simulink model "TwoLevel_ThreePhase_SVM_2017b"  (R2017b)
settings: Solver=VariableStepAuto  StartTime=0.0  StopTime=0.1  RelTol=1e-3
StopFcn:
  | Vabc=out.Vabc;
  | Vab=out.Vab;
  | Iabc=out.Iabc;
libraries: powerlib x12
settings Model: Creator=Mehdi  LastModifiedBy=Mehdi
settings DataIOCC: ReturnWorkspaceOutputs=on
settings DebuggingCC: UnconnectedInputMsg=none  UnconnectedOutputMsg=none  UnconnectedLineMsg=none
settings ModelReferenceCC: EnableRefExpFcnMdlSchedulingChecks=off
settings SFSimCC: SimUseLocalCustomCode=on
settings RTWCC: Description=Generic Real-Time Target  RTWUseLocalCustomCode=on
settings CodeAppCC: StateflowObjectComments=on
settings SimscapeCC: SimscapeNormalizeSystem=off

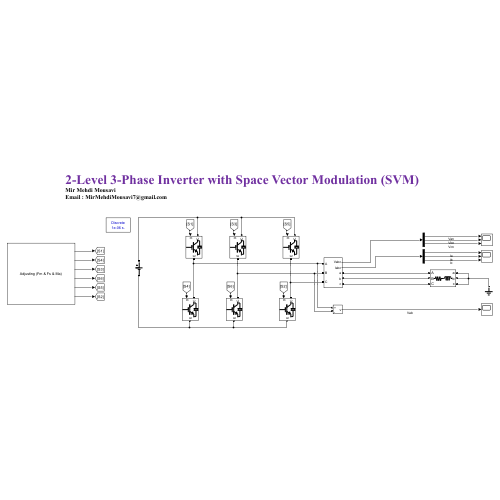
[thumbnail: Simulink's stored preview of the top-level diagram]
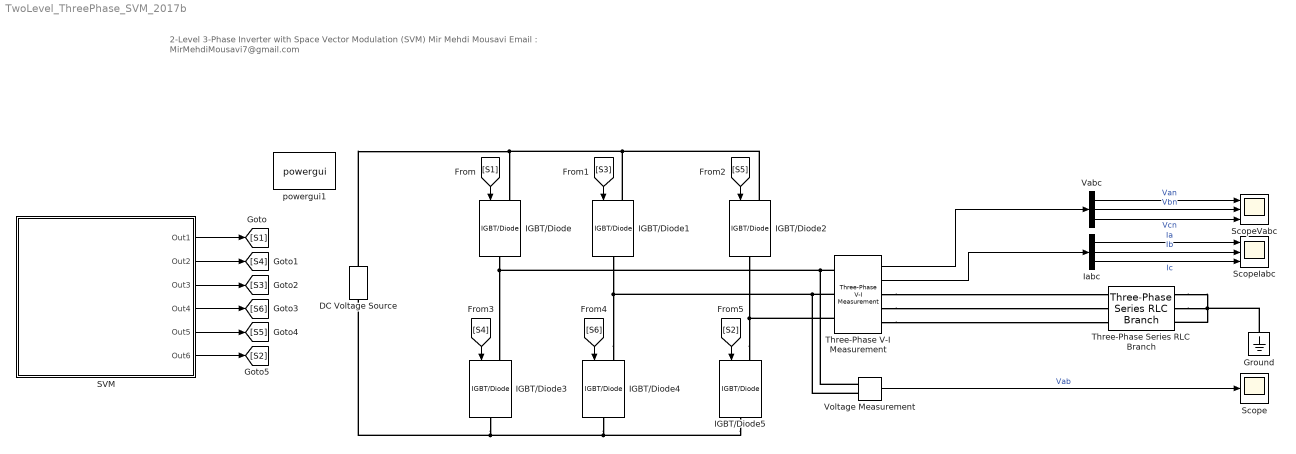
== system TwoLevel_ThreePhase_SVM_2017b ==
  note: 2-Level 3-Phase Inverter with Space Vector Modulation (SVM)
      | Mir Mehdi Mousavi
      | Email : MirMehdiMousavi7@gmail.com
  DC Voltage Source : powerlib/Electrical Sources/DC Voltage Source  Amplitude=400  Measurements=None
  Ground : powerlib/Elements/Ground  LConnTagsString=a
  IGBT/Diode{,1..5} (6 alike) : powerlib/Power Electronics/IGBT//Diode  Ron=1e-3  Rs=1e5  Cs=inf  Measurements=off
  Iabc : Demux  Outputs=3
  SVM : Subsystem  mask{f=50, m=1, fs=1750}
      mask prompts: f "Reference Frequency (Hz) :"; m "Modulation Index Ma :"; fs "Switching Frequency Fs :"
      mask Display: fprintf('Adjusting (Fm & Fs & Ma)' )
  Scope : Scope
  ScopeIabc : Scope  NumInputPorts=3
  ScopeVabc : Scope  NumInputPorts=3
  Three-Phase Series RLC Branch : powerlib/Elements/Three-Phase Series RLC Branch  LConnTagsString=A|B|C  RConnTagsString=A|B|C  BranchType=RL  Resistance=3  Inductance=1.5e-2  Capacitance=1e-6  Measurements=None
  Three-Phase V-I Measurement : powerlib/Measurements/Three-Phase V-I Measurement  VoltageMeasurement=phase-to-ground  SetLabelV=off  LabelV=Vabc  Vpu=off  VpuLL=off  CurrentMeasurement=yes  SetLabelI=off  LabelI=Iabc  Ipu=off  Pbase=100e6  Vbase=500e3  OutputType=Complex  PhasorSimulation=off  PSBequivalent=0
  Vabc : Demux  Outputs=3
  Voltage Measurement : powerlib/Measurements/Voltage Measurement  PhasorSimulation=off  OutputType=Complex  PSBequivalent=0
  powergui1 : powerlib/powergui  Priority=1  SimulationMode=Discrete  SampleTime=1e-6  frequency=60  Iterations=50  frequencyindice=0  Pbase=100e6  ErrMax=1e-4  UnitsV=kV  UnitsW=MW  buscounter=0  FunctionMessages=off  echomessages=off  EnableUseOfTLC=off  CurrentSourceSwitches=off  DisableSnubberDevices=off  DisableRonSwitches=off  DisableVfSwitches=off  DisplayEquations=off  AutomaticDiscreteSolvers=off  SolverType=Tustin/Backward Euler (TBE)  Interpol=off  ExternalGateDelay=off  methode=off  Ts=10  x0status=blocks  SPID=off  SwTol=0  HookPort=off  NonlinearTolerance=1e-4  nMaxIteration=100  ContinueOnMaxIteration=off  RestoreLinks=warning  ResistiveCurrentMeasurement=off  Frange=[0:2:500]  Ylog=off  Xlog=on  ShowGrid=off  save=off  variable=ZData  structure=0  ZoomFFT=off  StartTime=0.0  cycles=1  DisplayStyle=1  fundamental=60  FreqAxis=off  MaxFrequency=1000  frequencyindicesteady=1  RmsSteady=1  display=off
  wires:
  [S3] -> IGBT/Diode1/1
  Three-Phase V-I Measurement/1 -> Vabc/1
  [S6] -> IGBT/Diode4/1
  [S4] -> IGBT/Diode3/1
  [S2] -> IGBT/Diode5/1
  [S1] -> IGBT/Diode/1
  [S5] -> IGBT/Diode2/1
  Three-Phase V-I Measurement/2 -> Iabc/1
  Vabc/1 -> ScopeVabc/1  "Van"
  Vabc/2 -> ScopeVabc/2  "Vbn"
  Vabc/3 -> ScopeVabc/3  "Vcn"
  Iabc/1 -> ScopeIabc/1  "Ia"
  Iabc/2 -> ScopeIabc/2  "Ib"
  Iabc/3 -> ScopeIabc/3  "Ic"
  Voltage Measurement/1 -> Scope/1  "Vab"
  SVM/1(Out1) -> [S1]
  SVM/2(Out2) -> [S4]
  SVM/3(Out3) -> [S3]
  SVM/4(Out4) -> [S6]
  SVM/5(Out5) -> [S5]
  SVM/6(Out6) -> [S2]
  connections:
  IGBT/Diode4/LConn1 -- Voltage Measurement/LConn2 -- Three-Phase V-I Measurement/LConn2 -- IGBT/Diode1/RConn1
  IGBT/Diode2/LConn1 -- IGBT/Diode1/LConn1 -- DC Voltage Source/RConn1 -- IGBT/Diode/LConn1
  Three-Phase Series RLC Branch/RConn2 -- Ground/LConn1 -- Three-Phase Series RLC Branch/RConn1 -- Three-Phase Series RLC Branch/RConn3
  Three-Phase V-I Measurement/LConn1 -- Voltage Measurement/LConn1 -- IGBT/Diode/RConn1 -- IGBT/Diode3/LConn1
  IGBT/Diode5/LConn1 -- Three-Phase V-I Measurement/LConn3 -- IGBT/Diode2/RConn1
  DC Voltage Source/LConn1 -- IGBT/Diode3/RConn1 -- IGBT/Diode4/RConn1 -- IGBT/Diode5/RConn1
  Three-Phase V-I Measurement/RConn3 -- Three-Phase Series RLC Branch/LConn3
  Three-Phase V-I Measurement/RConn2 -- Three-Phase Series RLC Branch/LConn2
  Three-Phase V-I Measurement/RConn1 -- Three-Phase Series RLC Branch/LConn1

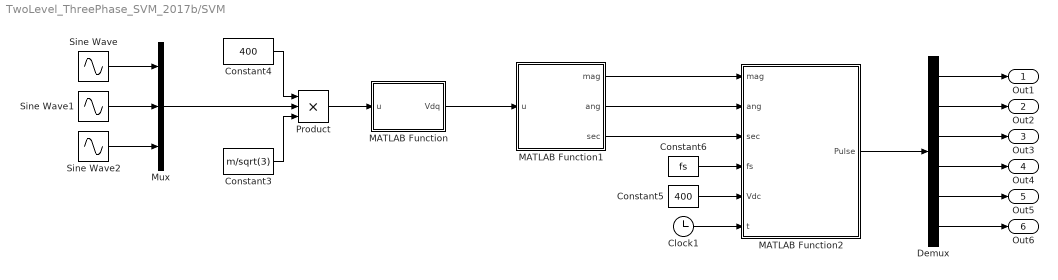
== system TwoLevel_ThreePhase_SVM_2017b/SVM ==
  Clock1 : Clock
  Constant3 : Constant  Value=m/sqrt(3)
  Constant4 : Constant  Value=400
  Constant5 : Constant  Value=400
  Constant6 : Constant  Value=fs
  Demux : Demux  Outputs=6
  MATLAB Function : MATLAB Function  TreatAsAtomicUnit=on
  MATLAB Function1 : MATLAB Function  TreatAsAtomicUnit=on
  MATLAB Function2 : MATLAB Function  TreatAsAtomicUnit=on
  Mux : Mux  Inputs=3
  Product : Product  Inputs=3
  Sine Wave : Sin  Frequency=2*pi*f  SampleTime=1e-6
  Sine Wave1 : Sin  Frequency=2*pi*f  Phase=4*pi/3  SampleTime=1e-6
  Sine Wave2 : Sin  Frequency=2*pi*f  Phase=2*pi/3  SampleTime=1e-6
  Out1 : Outport
  Out2 : Outport  Port=2
  Out3 : Outport  Port=3
  Out4 : Outport  Port=4
  Out5 : Outport  Port=5
  Out6 : Outport  Port=6
  wires:
  MATLAB Function/1(Vdq) -> MATLAB Function1/1(u)
  Sine Wave1/1 -> Mux/2
  Product/1 -> MATLAB Function/1(u)
  Sine Wave/1 -> Mux/1
  Sine Wave2/1 -> Mux/3
  Constant6/1 -> MATLAB Function2/4(fs)
  Constant4/1 -> Product/1
  Constant5/1 -> MATLAB Function2/5(Vdc)
  Demux/1 -> Out1/1
  MATLAB Function1/1(mag) -> MATLAB Function2/1(mag)
  Mux/1 -> Product/2
  Constant3/1 -> Product/3
  Demux/6 -> Out6/1
  MATLAB Function1/2(ang) -> MATLAB Function2/2(ang)
  MATLAB Function2/1(Pulse) -> Demux/1
  Clock1/1 -> MATLAB Function2/6(t)
  MATLAB Function1/3(sec) -> MATLAB Function2/3(sec)
  Demux/4 -> Out4/1
  Demux/2 -> Out2/1
  Demux/3 -> Out3/1
  Demux/5 -> Out5/1

== matlab function TwoLevel_ThreePhase_SVM_2017b/SVM/MATLAB Function1 ==
  data: u input; mag output; ang output; sec output
function [mag,ang,sec] = fcn(u)

z=u(1)+1i*u(2);

mag = abs(z);
ang = atan2(imag(z),real(z));

alpha= ang*180/pi;

sec = (alpha>0 & alpha<=60)*1 + (alpha>60 & alpha<=120)*2 + (alpha>120 & alpha<=180)*3 +(alpha>-180 & alpha<=-120)*4 +(alpha>-120 & alpha<=-60)*5 +(alpha>-60 & alpha<=0)*6 ;

== matlab function TwoLevel_ThreePhase_SVM_2017b/SVM/MATLAB Function ==
  data: u input; Vdq output
function Vdq = fcn(u)
Va=u(1);
Vb=u(2);
Vc=u(3);

Vd=(2/3)*(Va-0.5*Vb-0.5*Vc);
Vq=(2/3)*(0*Va+(sqrt(3)/2)*Vb-(sqrt(3)/2)*Vc);

Vdq=[Vd;Vq];

== matlab function TwoLevel_ThreePhase_SVM_2017b/SVM/MATLAB Function2 ==
  data: mag input; ang input; sec input; fs input; Vdc input; t input; Pulse output
function Pulse  = fcn(mag,ang,sec,fs,Vdc,t)

m=sqrt(3)*(mag/Vdc);
Ta=m*sin(sec*pi/3 -ang)/fs;
Tb=m*sin(ang - ((sec-1)*pi/3))/fs;
T0= (1/fs - Ta - Tb);

odd_sec=mod(floor(sec),2);
if(odd_sec~=1)  
    
 Ta=m*sin(ang - ((sec-1)*pi/3))/fs;
 Tb=m*sin(sec*pi/3 - ang)/fs;
 
end

ref= rem(t,1/fs); 

int1=T0/4;
int2=int1+Ta/2;
int3=int2+Tb/2;
int4=int3+T0/2;
int5=int4+Tb/2;
int6=int5+Ta/2;

time_int=1+(ref>=int1)+(ref>=int2)+(ref>=int3)+(ref>=int4)+(ref>=int5)+(ref>=int6);

sw_state=zeros(3,7,6);  

sw_state(:,:,1)=[0	1	1	1	1	1	0;0  0	1	1	1	0	0; 0	0	0	1	0	0	0]; %sector 1
sw_state(:,:,2)=[0	0	1	1	1	0	0;0	 1	1	1	1	1	0; 0	0	0	1	0	0	0]; %sector 2
sw_state(:,:,3)=[0	0	0	1	0	0	0;0	 1	1	1	1	1	0; 0	0	1	1	1	0	0]; %sector 3
sw_state(:,:,4)=[0	0	0	1	0	0	0;0	 0	1	1	1	0	0; 0	1	1	1	1	1	0]; %sector 4
sw_state(:,:,5)=[0	0	1	1	1	0	0;0	 0	0	1	0	0	0; 0	1	1	1	1	1	0]; %sector 5
sw_state(:,:,6)=[0	1	1	1	1	1	0;0	 0	0	1	0	0	0; 0	0	1	1	1	0	0]; %sector 6

if t<100e-6
sec=1;
end;

S1=sw_state(1,time_int,sec);
S2= ~S1;
S3=sw_state(2,time_int,sec);
S4= ~S3;
S5=sw_state(3,time_int,sec);
S6= ~S5;

Pulse= [S1 S2 S3 S4 S5 S6];

end
